simulink model "speedgoat_complete_1GDL_model"  (R2023b)
settings: Solver=FixedStepAuto  StartTime=0.0  StopTime=inf  FixedStep=0.001  RelTol=1e-3  EnableMultiTasking=on
undefined symbols (not defined in the file): hems, IO316, IO3xx, m
libraries: speedgoatlib_IO110 x2, speedgoatlib_fpga_pwm x1, speedgoatlib_fpga x1
settings Model: Creator=ricardo  LastModifiedBy=ricardo
settings SolverCC: ConcurrentTasks=on  AlgebraicLoopSolver=TrustRegion  PositivePriorityOrder=on  InsertRTBMode=Never (minimum delay)
settings DataIOCC: SaveFormat=Array  SaveState=on  SignalLoggingName=logsOut
settings OptimizationCC: BlockReduction=off  BooleanDataType=off  OptimizeBlockIOStorage=off  BufferReuse=off  ReuseModelBlockBuffer=off  GlobalBufferReuse=off  ExpressionFolding=off  LocalBlockOutputs=off  InitFltsAndDblsToZero=on  OptimizeDataStoreBuffers=off  BusAssignmentInplaceUpdate=off
settings DebuggingCC: SaveWithParameterizedLinksMsg=none  UnderspecifiedInitializationDetection=Classic  MergeDetectMultiDrivingBlocksExec=none  CheckExecutionContextPreStartOutputMsg=on  SignalResolutionControl=TryResolveAllWithWarning  TasksWithSamePriorityMsg=none  UnconnectedInputMsg=warning  UnconnectedOutputMsg=warning  UnconnectedLineMsg=warning  SFUnexpectedBacktrackingDiag=warning  SFNoUnconditionalDefaultTransitionDiag=warning  SFExecutionAtInitializationDiag=none  ArithmeticOperatorsInVariantConditions=warning
settings HardwareCC: ProdBitPerLong=64  ProdLongLongMode=on  ProdHWDeviceType=Intel->x86-64 (Linux 64)
settings ModelReferenceCC: EnableRefExpFcnMdlSchedulingChecks=on  PropagateSignalLabelsOutOfModel=off
settings SFSimCC: SimUseLocalCustomCode=off  SimTargetLang=C++
settings RTWCC: Description=Simulink Real-Time  SystemTargetFile=slrealtime.tlc  TemplateMakefile=slrealtime_default_tmf  RTWUseLocalCustomCode=off  Toolchain=Simulink Real-Time Toolchain  BuildConfiguration=Faster Runs  CodeExecutionProfiling=on  TargetLang=C++  DLArmComputeVersion=19.05
settings CodeAppCC: StateflowObjectComments=on
settings SimulinkRealTimeTargetCC: MATLABClassNameForMDSCustomization=Simulink.SoftwareTarget.GRTCustomization  UseGCCFastMath=on
settings ConfigComp: CovMetricSettings=dw  CovSaveCumulativeToWorkspaceVar=on  CovSaveSingleToWorkspaceVar=on  CovExternalEMLEnable=off  CovSFcnEnable=off

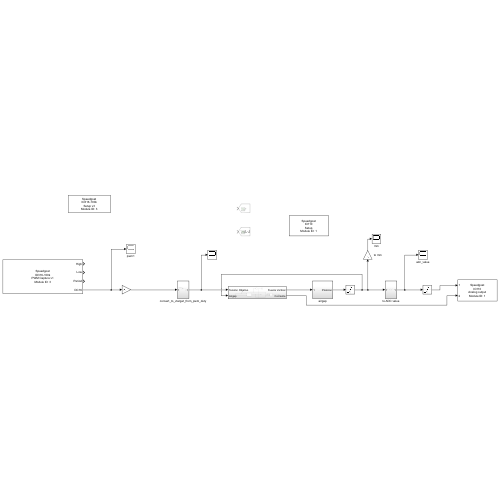
[thumbnail: Simulink's stored preview of the top-level diagram]
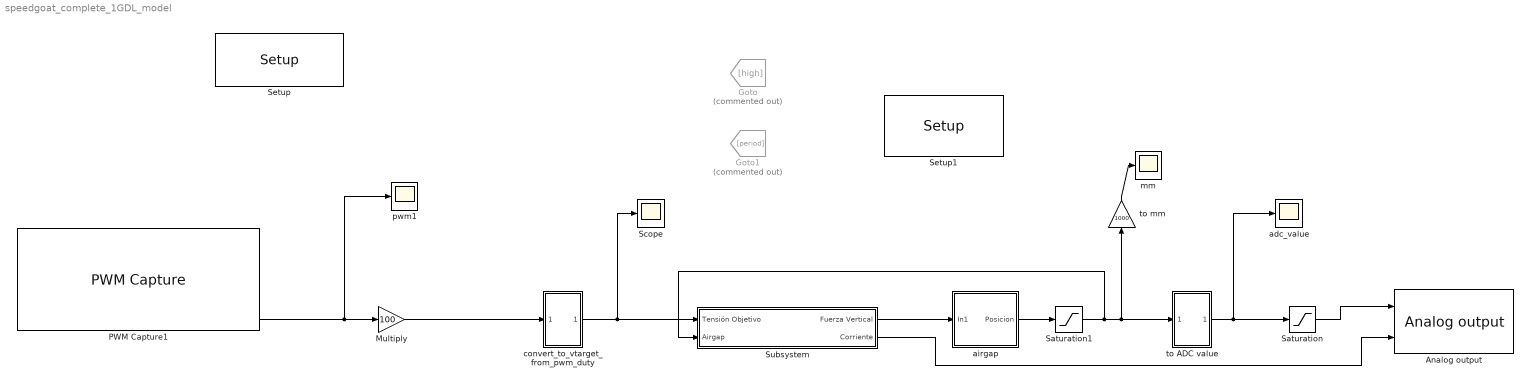
== system speedgoat_complete_1GDL_model ==
  Analog output : speedgoatlib_IO110/Analog output  id=1  ts=0.001  channels=[1,2]  range=[0,0,0,0,4,4,4,4,4,4,4,4,4,4,4,4,4,4,4,4,4,4,4,4,4,4,4,4,4,4,4,4]  pciSlot=-1  init=[0,0]  reset=[1,1]
      settings: SourceProductName=Simulink Real-Time: Speedgoat I/O Blockset
  Goto : Goto  Commented=on  GotoTag=high
  Goto1 : Goto  Commented=on  GotoTag=period
  Multiply : Gain  Gain=100
  PWM Capture1 : speedgoatlib_fpga_pwm/PWM Capture  id=3  chan=[34]  ts=0.001  enableDma=on  captureMode=High transitions triggered  bit_width_cap=24  captureTimeout_si=0  captureTimeout_eff=0  captureTimeout=0  debounce_si=10e-6  debounce_eff=10e-6  debounce=750  showHighDuration=on  showLowDuration=on  showPeriod=on  showDC16=on  showDC8=off  showTOn=off  showTOff=off  showValidData=off
      settings: SourceProductName=Simulink Real-Time: Speedgoat I/O Blockset
  Saturation : Saturate  UpperLimit=3.3  LowerLimit=0
  Saturation1 : Saturate  UpperLimit=0.0225  LowerLimit=0.009
  Scope : Scope
  Setup : speedgoatlib_fpga/Setup/Setup  board=IO316-100k  id=3  device_id=1  frontIO=None  rearIO=IO3xx-21  bitstreamFile=speedgoat_IO316_100k_21_CI_02826_v1  rev=1.000000  timestamp_string=25/03/24 14:47:22  fpgaFreq=75 MHz  fpgaTick=13.33 ns  ProgSpiFlash=off  ProgBPIFlash=off  pciSlot=-1  useFpgaDmaController=off  PullRPort0=pull-up 3.3V  VioPort0=3.3V  PullRPort1=pull-up 3.3V  VioPort1=3.3V  PullRPort2=pull-up 3.3V  VioPort2=3.3V  PullRPort3=pull-up 3.3V  VioPort3=3.3V  PullRPort4=pull-up 3.3V  VioPort4=3.3V  PullRPort5=pull-up 3.3V  VioPort5=3.3V  PullRPort6=pull-up 3.3V  VioPort6=3.3V  diffLineTermination_rear1=on  diffLineTermination_rear2=on  diffLineTermination_rear3=on  diffLineTermination_rear4=on  diffLineTermination_rear5=on  diffLineTermination_rear6=on  diffLineTermination_rear7=on  diffLineTermination_rear8=on  PullRPort15=pull-up 3.3V  PullRPort31=pull-up 3.3V  PullRPort47=pull-up 3.3V  PullRPort63=pull-up 3.3V  diffLineTermination_1=on  diffLineTermination_2=on  diffLineTermination_3=on  diffLineTermination_4=on  diffLineTermination_5=on  diffLineTermination_6=on  diffLineTermination_7=on  diffLineTermination_8=on  diffLineTermination_9=on  diffLineTermination_10=on  diffLineTermination_11=on  diffLineTermination_12=on  diffLineTermination_13=on  diffLineTermination_14=on  diffLineTermination_15=on  diffLineTermination_16=on  diffLineTermination_17=on  diffLineTermination_18=on  diffLineTermination_19=on  diffLineTermination_20=on  diffLineTermination_21=on  diffLineTermination_22=on  diffLineTermination_23=on  diffLineTermination_24=on  diffLineTermination_25=on  diffLineTermination_26=on  diffLineTermination_27=on  diffLineTermination_28=on  diffLineTermination_29=on  diffLineTermination_30=on  diffLineTermination_31=on  diffLineTermination_32=on  Vo_36x_1=3.3V  Vi_Pull_36x_1=Floating  Vo_36x_2=3.3V  Vi_Pull_36x_2=Floating  Vo_36x_3=3.3V  Vi_Pull_36x_3=Floating  Vo_36x_4=3.3V  Vi_Pull_36x_4=Floating  Vo_36x_5=3.3V  Vi_Pull_36x_5=Floating  Vo_36x_6=3.3V  Vi_Pull_36x_6=Floating  Vo_36x_7=3.3V  Vi_Pull_36x_7=Floating  Vo_36x_8=3.3V  Vi_Pull_36x_8=Floating  Vo_36x_9_16=3.3V  Vi_Pull_36x_9_16=Floating  Vo_36x_17_24=3.3V  Vi_Pull_36x_17_24=Floating  Vo_36x_25_32=3.3V  Vi_Pull_36x_25_32=Floating  Vo_36x_33_40=3.3V  Vi_Pull_36x_33_40=Floating  Vo_36x_41_48=3.3V  Vi_Pull_36x_41_48=Floating  Vo_36x_49_56=3.3V  Vi_Pull_36x_49_56=Floating  Vo_36x_57_64=3.3V  Vi_Pull_36x_57_64=Floating
      settings: SourceProductName=Simulink Real-Time: Speedgoat I/O Blockset
  Setup1 : speedgoatlib_IO110/Setup  group=Module setup  id=1  daChannel=[1,2]  daInitValue=[0]  daReset=[1]  pciSlot=-1  daRange00=0V .. 5V  daRange01=0V .. 5V  daRange02=0V .. 5V  daRange03=0V .. 5V  daTSD0=off  daClamp0=on  daRange10=-10V .. +10V  daRange11=-10V .. +10V  daRange12=-10V .. +10V  daRange13=-10V .. +10V  daTSD1=off  daClamp1=on  daRange20=-10V .. +10V  daRange21=-10V .. +10V  daRange22=-10V .. +10V  daRange23=-10V .. +10V  daTSD2=off  daClamp2=on  daRange30=-10V .. +10V  daRange31=-10V .. +10V  daRange32=-10V .. +10V  daRange33=-10V .. +10V  daTSD3=off  daClamp3=on  daRange40=-10V .. +10V  daRange41=-10V .. +10V  daRange42=-10V .. +10V  daRange43=-10V .. +10V  daTSD4=off  daClamp4=on  daRange50=-10V .. +10V  daRange51=-10V .. +10V  daRange52=-10V .. +10V  daRange53=-10V .. +10V  daTSD5=off  daClamp5=on  daRange60=-10V .. +10V  daRange61=-10V .. +10V  daRange62=-10V .. +10V  daRange63=-10V .. +10V  daTSD6=off  daClamp6=on  daRange70=-10V .. +10V  daRange71=-10V .. +10V  daRange72=-10V .. +10V  daRange73=-10V .. +10V  daTSD7=off  daClamp7=on
      settings: SourceProductName=Simulink Real-Time: Speedgoat I/O Blockset
  Subsystem : Subsystem
  adc_value : Scope
  airgap : Subsystem
  convert_to_vtarget_from_pwm_duty : Subsystem
  mm : Scope
  pwm1 : Scope
  to ADC value : Subsystem
  to mm : Gain  Gain=1000
  wires:
  convert_to_vtarget_from_pwm_duty/1(Out1) -> Scope/1, Subsystem/1(Tensión Objetivo)
  Saturation/1 -> Analog output/1
  Saturation1/1 -> to mm/1, to ADC value/1(In1), Subsystem/2(Airgap)
  airgap/1(Posicion) -> Saturation1/1
  Multiply/1 -> convert_to_vtarget_from_pwm_duty/1(In1)
  to ADC value/1(Out1) -> adc_value/1, Saturation/1
  Subsystem/1(Fuerza Vertical) -> airgap/1(In1)
  to mm/1 -> mm/1
  PWM Capture1/4 -> pwm1/1, Multiply/1
  Subsystem/2(Corriente) -> Analog output/2

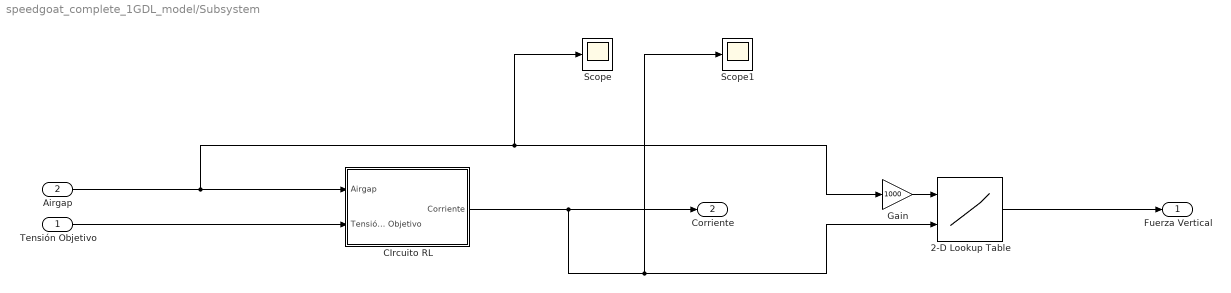
== system speedgoat_complete_1GDL_model/Subsystem ==
  Tensión Objetivo : Inport
  Airgap : Inport  Port=2
  2-D Lookup Table : Lookup_n-D  BreakpointsForDimension1=hems.Airgap  BreakpointsForDimension2=hems.Current  Table=hems.Force_Vertical  InternalRulePriority=Speed  RndMeth=Simplest
      settings: InputPortMap=u0,u1
  CIrcuito RL : Subsystem
  Gain : Gain  Gain=1000
  Scope : Scope
  Scope1 : Scope
  Fuerza Vertical : Outport
  Corriente : Outport  Port=2
  wires:
  Tensión Objetivo/1 -> CIrcuito RL/2(Tensión Objetivo)
  2-D Lookup Table/1 -> Fuerza Vertical/1
  Gain/1 -> 2-D Lookup Table/1
  Airgap/1 -> Scope/1, Gain/1, CIrcuito RL/1(Airgap)
  CIrcuito RL/1(Corriente) -> Corriente/1, Scope1/1, 2-D Lookup Table/2

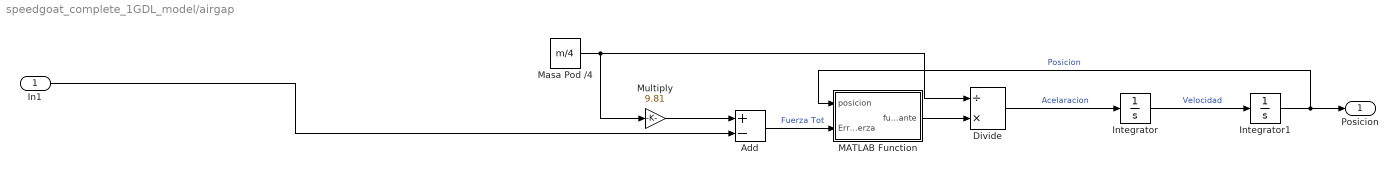
== system speedgoat_complete_1GDL_model/airgap ==
  In1 : Inport
  Add : Sum  Inputs=+-
  Divide : Product  Inputs=/*
  Integrator : Integrator
  Integrator1 : Integrator  InitialCondition=0.0225
  MATLAB Function : MATLAB Function  TreatAsAtomicUnit=on
  Masa Pod /4 : Constant  Value=m/4
  Multiply : Gain  Gain=9.81
  Posicion : Outport
  wires:
  Multiply/1 -> Add/1
  Masa Pod /4/1 -> Divide/1, Multiply/1
  MATLAB Function/1(fuerza_resultante) -> Divide/2
  Divide/1 -> Integrator/1  "Acelaracion"
  Integrator/1 -> Integrator1/1  "Velocidad"
  Add/1 -> MATLAB Function/2(Error_fuerza)  "Fuerza Tot"
  In1/1 -> Add/2
  Integrator1/1 -> Posicion/1, MATLAB Function/1(posicion)  "Posicion"

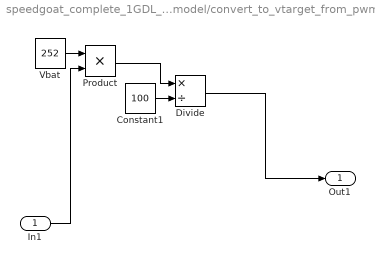
== system speedgoat_complete_1GDL_model/convert_to_vtarget_from_pwm_duty ==
  In1 : Inport
  Constant1 : Constant  Value=100
  Divide : Product  Inputs=*/
  Product : Product
  Vbat : Constant  Value=252
  Out1 : Outport
  wires:
  Product/1 -> Divide/1
  Constant1/1 -> Divide/2
  In1/1 -> Product/2
  Vbat/1 -> Product/1
  Divide/1 -> Out1/1

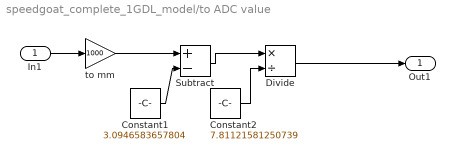
== system speedgoat_complete_1GDL_model/to ADC value ==
  In1 : Inport
  Constant1 : Constant  Value=3.0946583657804
  Constant2 : Constant  Value=7.81121581250739
  Divide : Product  Inputs=*/
  Subtract : Sum  Inputs=+-
  to mm : Gain  Gain=1000
  Out1 : Outport
  wires:
  In1/1 -> to mm/1
  Subtract/1 -> Divide/1
  Constant1/1 -> Subtract/2
  Divide/1 -> Out1/1
  to mm/1 -> Subtract/1
  Constant2/1 -> Divide/2

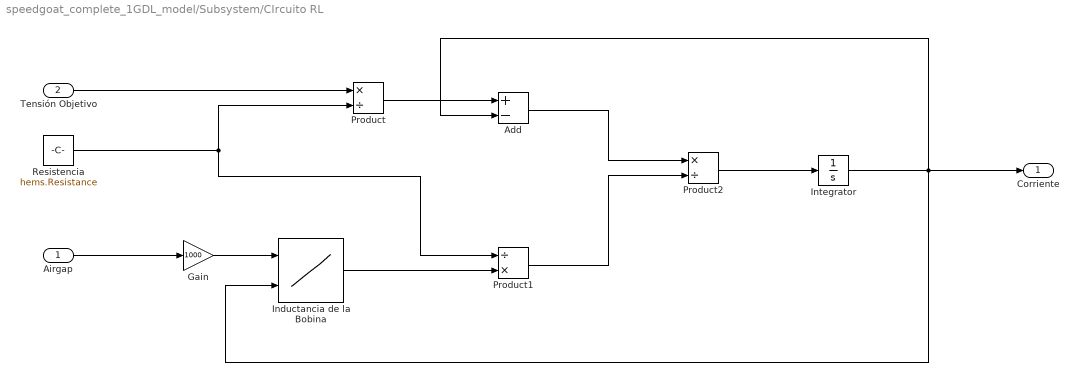
== system speedgoat_complete_1GDL_model/Subsystem/CIrcuito RL ==
  Airgap : Inport
  Tensión Objetivo : Inport  Port=2
  Add : Sum  Inputs=+-
  Gain : Gain  Gain=1000
  Inductancia de la Bobina : Lookup_n-D  BreakpointsForDimension1=hems.Airgap  BreakpointsForDimension2=hems.Current(1:109)  Table=hems.Inductance  InternalRulePriority=Speed  RndMeth=Simplest
      settings: InputPortMap=u0,u1
  Integrator : Integrator
  Product : Product  Inputs=*/
  Product1 : Product  Inputs=/*
  Product2 : Product  Inputs=*/
  Resistencia : Constant  Value=hems.Resistance
  Corriente : Outport
  wires:
  Inductancia de la Bobina/1 -> Product1/2
  Product1/1 -> Product2/2
  Product/1 -> Add/1
  Resistencia/1 -> Product1/1, Product/2
  Airgap/1 -> Gain/1
  Integrator/1 -> Corriente/1, Inductancia de la Bobina/2, Add/2
  Add/1 -> Product2/1
  Product2/1 -> Integrator/1
  Tensión Objetivo/1 -> Product/1
  Gain/1 -> Inductancia de la Bobina/1

== matlab function speedgoat_complete_1GDL_model/airgap/MATLAB Function ==
  data: posicion input; Error_fuerza input; fuerza_resultante output
function fuerza_resultante = fcn(posicion, Error_fuerza) %Siendo Error_fuerza= Fg-FHems

if posicion > 0.0225

    if Error_fuerza >= 0

    fuerza_resultante = Error_fuerza - (62.5*9.81); % Fg-FHems-Fg --> N=Fg

    else                                            %En este caso N = 0

     fuerza_resultante = Error_fuerza;

    end

else

    fuerza_resultante = Error_fuerza;

end

end
